simulink model "model_PD"  (R2016b)
settings: Solver=VariableStepAuto  StartTime=0.0  StopTime=30  FixedStep=Ts  RelTol=1e-3  EnableMultiTasking=on
values from neighbouring files (symbols this model uses):
  C = [eye(3),zeros(3,9);zeros(3,6),eye(3),zeros(3,3);zeros(3,9),eye(3)]    [model_script_Cascade.m]    (also in model_script_LQR_LQI.m; model_script_PD.m)
  D_height = .6117    (= 0.6117)    [model_script_Cascade.m]    (also in model_script_PD.m)
  D_pitch = .2256    (= 0.2256)    [model_script_Cascade.m]    (also in model_script_PD.m)
  D_roll = 0.1522    [model_script_Cascade.m]    (also in model_script_PD.m)
  D_yaw = .0367    (= 0.0367)    [model_script_Cascade.m]    (also in model_script_PD.m)
  g = 9.81    [model_script_Cascade.m]    (also in model_script_LQR_LQI.m; model_script_PD.m)
  I = diag([Ixx;Iyy;Izz])    [model_script_Cascade.m]    (also in model_script_LQR_LQI.m; model_script_PD.m)
  i0 = [tauphi;tautheta;taupsi;T]    [model_script_Cascade.m]    (also in model_script_LQR_LQI.m; model_script_PD.m)
  M = 0.487    [model_script_Cascade.m]    (also in model_script_LQR_LQI.m; model_script_PD.m)
  mean_att = zeros(3,1)    [model_script_Cascade.m]    (also in model_script_LQR_LQI.m; model_script_PD.m)
  mean_av = zeros(3,1)    [model_script_Cascade.m]    (also in model_script_LQR_LQI.m; model_script_PD.m)
  mean_pos = zeros(3,1)    [model_script_Cascade.m]    (also in model_script_LQR_LQI.m; model_script_PD.m)
  P_height = .3843    (= 0.3843)    [model_script_Cascade.m]    (also in model_script_PD.m)
  P_pitch = 1.9491    [model_script_Cascade.m]    (also in model_script_PD.m)
  P_roll = 1.5117    [model_script_Cascade.m]    (also in model_script_PD.m)
  P_yaw = .1152    (= 0.1152)    [model_script_Cascade.m]    (also in model_script_PD.m)
  propDistance = 0.125    [model_script_Cascade.m]    (also in model_script_LQR_LQI.m; model_script_PD.m)
  Q = diag([1e-5,1e-5,1e-5,1e-7,1e-7,1e-4,ones(1,2)*2e-7,6e-7,ones(1,3)*1e-7])    [model_script_Cascade.m]    (also in model_script_LQR_LQI.m; model_script_PD.m)
  R = diag(var)    [model_script_Cascade.m]    (also in model_script_LQR_LQI.m; model_script_PD.m)
  T_att = 1/200    (= 0.005)    [model_script_Cascade.m]    (also in model_script_LQR_LQI.m; model_script_PD.m)
  T_xy = 1/10    (= 0.1)    [model_script_Cascade.m]    (also in model_script_LQR_LQI.m; model_script_PD.m)
  T_yaw = 1/100    (= 0.01)    [model_script_Cascade.m]    (also in model_script_LQR_LQI.m; model_script_PD.m)
  T_z = 1/25    (= 0.04)    [model_script_Cascade.m]    (also in model_script_LQR_LQI.m; model_script_PD.m)
  var_att = [9.44454290406988e-06 1.41319492944844e-05 0.000590278082576831]'    [model_script_Cascade.m]    (also in model_script_LQR_LQI.m; model_script_PD.m)
  var_av = [8.38442613623844e-07 9.65548247114005e-07 1.06378940883219e-06]'    [model_script_Cascade.m]    (also in model_script_LQR_LQI.m; model_script_PD.m)
  var_pos = ones(3,1)*0.00219628793119666    [model_script_Cascade.m]    (also in model_script_LQR_LQI.m; model_script_PD.m)
  xi0 = [x;y;z;u;v;w;phi;theta;psi;p;q;r]    [model_script_Cascade.m]    (also in model_script_LQR_LQI.m; model_script_PD.m)
  yawTorqueC = 5    [model_script_Cascade.m]    (also in model_script_LQR_LQI.m; model_script_PD.m)
undefined symbols (not defined in the file or in its folder): den_phi_d, den_theta_d, den_z_d, num_phi_d, num_theta_d, num_z_d, sigbuilder_block, T_pos
undefined symbols (not defined in the file): dronePowerScaling
libraries: aerolibutil x2, simulink x2
(part 1 of 2)
settings Model: Creator=Patrick  LastModifiedBy=s122802
settings OptimizationCC: LifeSpan=inf
settings DebuggingCC: SFUnexpectedBacktrackingDiag=warning  SFNoUnconditionalDefaultTransitionDiag=warning  SFExecutionAtInitializationDiag=none
settings GRTTargetCC: TargetLangStandard=C89/C90 (ANSI)  GeneratePreprocessorConditionals=Disable all
settings ConfigComp: CovMetricSettings=dw  CovHtmlReporting=on  CovSaveCumulativeToWorkspaceVar=on  CovSaveSingleToWorkspaceVar=on  CovExternalEMLEnable=off

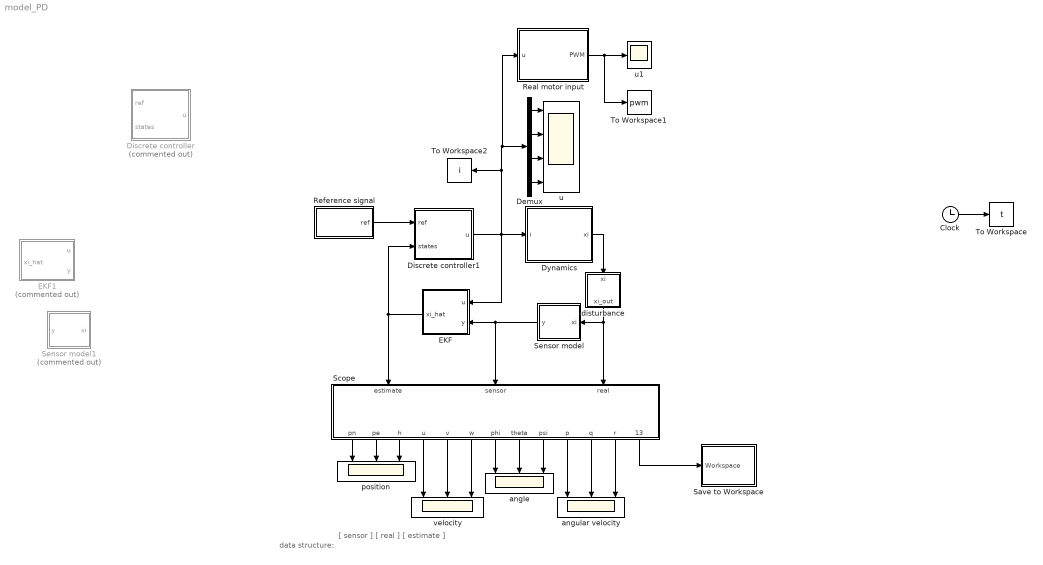
== system model_PD ==
  note: data structure:
  note: [ sensor   	]
      | [ real		]
      | [ estimate	]
  Clock : Clock
  Demux : Demux
  Discrete controller : Subsystem  Commented=on
  Discrete controller1 : Subsystem
  Dynamics : Subsystem
  EKF : Subsystem
  EKF1 : Subsystem  Commented=on
  Real motor input : Subsystem
  Reference signal : Subsystem
  Save to Workspace : Subsystem
  Scope : Subsystem
  Sensor model : Subsystem
  Sensor model1 : Subsystem  Commented=on
  To Workspace : ToWorkspace  VariableName=t  SampleTime=-1
      settings: Decimation=10
  To Workspace1 : ToWorkspace  VariableName=pwm  SampleTime=-1
      settings: Decimation=10
  To Workspace2 : ToWorkspace  VariableName=i  SampleTime=-1
      settings: Decimation=10
  angle : Scope  NumInputPorts=3
  angular velocity : Scope  NumInputPorts=3
  disturbance : Subsystem
  position : Scope  NumInputPorts=3
  u : Scope  NumInputPorts=4
  u1 : Scope
  velocity : Scope  NumInputPorts=3
  wires:
  Reference signal/1(ref) -> Discrete controller1/1(ref)
  Sensor model/1(y) -> EKF/2(y), Scope/2(sensor)
  Scope/2(pe) -> position/2
  Scope/10(p) -> angular velocity/1
  Scope/6(w) -> velocity/3
  Scope/5(v) -> velocity/2
  Scope/1(pn) -> position/1
  Scope/8(theta) -> angle/2
  Scope/9(psi) -> angle/3
  Scope/4(u) -> velocity/1
  Scope/11(q) -> angular velocity/2
  Scope/12(r) -> angular velocity/3
  Scope/3(h) -> position/3
  Dynamics/1(xi) -> disturbance/1(xi)
  EKF/1(xi_hat) -> Discrete controller1/2(states), Scope/1(estimate)
  Scope/13(Workspace) -> Save to Workspace/1(Workspace)
  Demux/1 -> u/1
  Demux/2 -> u/2
  Demux/3 -> u/3
  Demux/4 -> u/4
  Discrete controller1/1(u) -> EKF/1(u), To Workspace2/1, Real motor input/1(u), Demux/1, Dynamics/1(i)
  Scope/7(phi) -> angle/1
  disturbance/1(xi_out) -> Sensor model/1(xi), Scope/3(real)
  Real motor input/1(PWM) -> To Workspace1/1, u1/1
  Clock/1 -> To Workspace/1

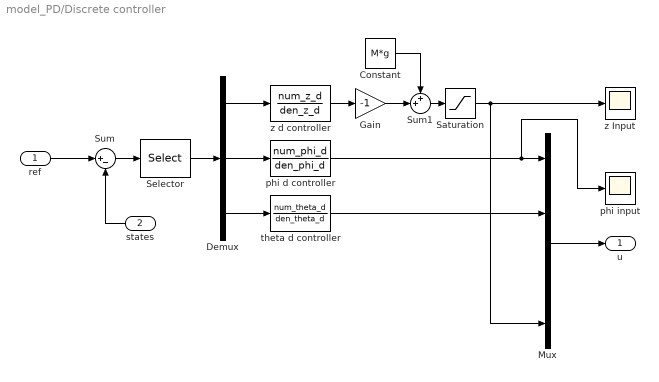
== system model_PD/Discrete controller ==
  ref : Inport
  states : Inport  Port=2
  Constant : Constant  Value=M*g
  Demux : Demux  Outputs=3
  Gain : Gain  Gain=-1
  Mux : Mux
  Saturation : Saturate  UpperLimit=10  LowerLimit=-10
  Selector : Selector  InputPortWidth=12  IndexOptions=Index vector (dialog)  Indices=[3 7 8]  OutputSizes=1
  Sum : Sum  Inputs=|+-
  Sum1 : Sum  Inputs=++|
  phi d controller : DiscreteTransferFcn  Numerator=num_phi_d  Denominator=den_phi_d
  phi input : Scope
  theta d controller : DiscreteTransferFcn  Numerator=num_theta_d  Denominator=den_theta_d
  z Input : Scope
  "z d controller " : DiscreteTransferFcn  Numerator=num_z_d  Denominator=den_z_d
  u : Outport
  wires:
  Demux/2 -> phi d controller/1
  Gain/1 -> Sum1/2
  Constant/1 -> Sum1/1
  Sum1/1 -> Saturation/1
  Selector/1 -> Demux/1
  Sum/1 -> Selector/1
  Demux/3 -> theta d controller/1
  Saturation/1 -> Mux/4, z Input/1
  "z d controller "/1 -> Gain/1
  theta d controller/1 -> Mux/2
  phi d controller/1 -> Mux/1, phi input/1
  states/1 -> Sum/2
  ref/1 -> Sum/1
  Demux/1 -> "z d controller "/1
  Mux/1 -> u/1

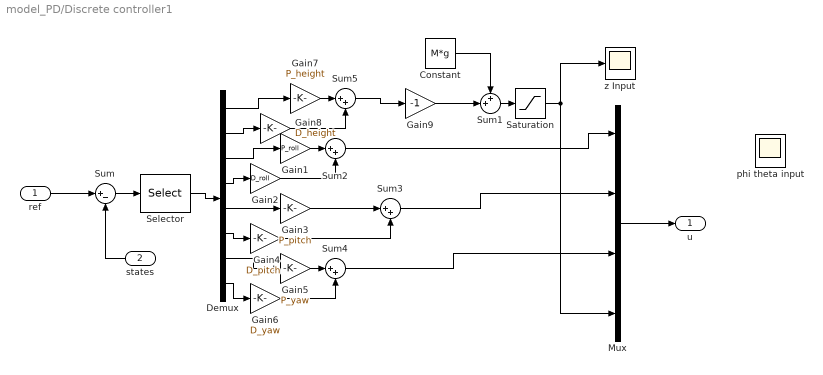
== system model_PD/Discrete controller1 ==
  ref : Inport
  states : Inport  Port=2
  Constant : Constant  Value=M*g
  Demux : Demux  Outputs=8
  Gain1 : Gain  Gain=P_roll
  Gain2 : Gain  Gain=D_roll
  Gain3 : Gain  Gain=P_pitch
  Gain4 : Gain  Gain=D_pitch
  Gain5 : Gain  Gain=P_yaw
  Gain6 : Gain  Gain=D_yaw
  Gain7 : Gain  Gain=P_height
  Gain8 : Gain  Gain=D_height
  Gain9 : Gain  Gain=-1
  Mux : Mux
  Saturation : Saturate  UpperLimit=10  LowerLimit=-10
  Selector : Selector  InputPortWidth=12  IndexOptions=Index vector (dialog)  Indices=[3 6 7 10 8 11 9 12]  OutputSizes=1
  Sum : Sum  Inputs=|+-
  Sum1 : Sum  Inputs=++|
  Sum{2..5} (4 alike) : Sum  Inputs=|++
  phi theta input : Scope  NumInputPorts=2
  z Input : Scope
  u : Outport
  wires:
  Mux/1 -> u/1
  ref/1 -> Sum/1
  states/1 -> Sum/2
  Sum3/1 -> Mux/2
  Saturation/1 -> Mux/4, z Input/1
  Sum/1 -> Selector/1
  Selector/1 -> Demux/1
  Sum1/1 -> Saturation/1
  Constant/1 -> Sum1/1
  Sum2/1 -> Mux/1
  Sum5/1 -> Gain9/1
  Gain5/1 -> Sum4/1
  Sum4/1 -> Mux/3
  Gain6/1 -> Sum4/2
  Gain2/1 -> Sum2/2
  Gain4/1 -> Sum3/2
  Gain1/1 -> Sum2/1
  Gain3/1 -> Sum3/1
  Demux/3 -> Gain1/1
  Demux/4 -> Gain2/1
  Demux/5 -> Gain3/1
  Demux/6 -> Gain4/1
  Demux/7 -> Gain5/1
  Demux/8 -> Gain6/1
  Gain8/1 -> Sum5/2
  Gain7/1 -> Sum5/1
  Demux/1 -> Gain7/1
  Demux/2 -> Gain8/1
  Gain9/1 -> Sum1/2

== system model_PD/Dynamics ==
  i : Inport
  Dynamics : Subsystem
  Mux : Mux
  xi : Outport
  wires:
  Mux/1 -> xi/1
  i/1 -> Dynamics/1(i)
  Dynamics/1(x y z) -> Mux/1
  Dynamics/2(u v w) -> Mux/2
  Dynamics/3(phi theta psi) -> Mux/3
  Dynamics/4(p q r) -> Mux/4

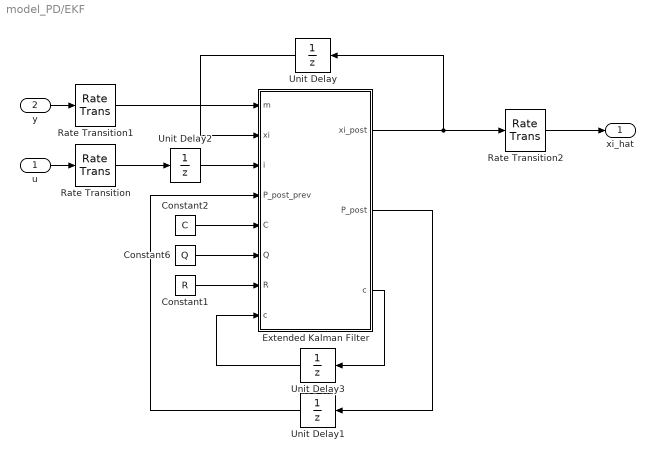
== system model_PD/EKF ==
  u : Inport
  y : Inport  Port=2
  Constant1 : Constant  Value=R
  Constant2 : Constant  Value=C
  Constant6 : Constant  Value=Q
  Extended Kalman Filter : MATLAB Function  TreatAsAtomicUnit=on
  Rate Transition : RateTransition  OutPortSampleTime=Ts
  Rate Transition1 : RateTransition  OutPortSampleTime=Ts
  Rate Transition2 : RateTransition  OutPortSampleTime=Ts
  Unit Delay : UnitDelay  InitialCondition=xi0  SampleTime=-1
  Unit Delay1 : UnitDelay  InitialCondition=zeros(12,12)  SampleTime=-1
  Unit Delay2 : UnitDelay  InitialCondition=i0  SampleTime=-1
  Unit Delay3 : UnitDelay  SampleTime=-1
  xi_hat : Outport
  wires:
  Extended Kalman Filter/3(c) -> Unit Delay3/1
  y/1 -> Rate Transition1/1
  Unit Delay3/1 -> Extended Kalman Filter/8("c ")
  Rate Transition2/1 -> xi_hat/1
  Rate Transition1/1 -> Extended Kalman Filter/1(m)
  Rate Transition/1 -> Unit Delay2/1
  u/1 -> Rate Transition/1
  Unit Delay2/1 -> Extended Kalman Filter/3(i)
  Unit Delay/1 -> Extended Kalman Filter/2(xi)
  Constant1/1 -> Extended Kalman Filter/7(R)
  Extended Kalman Filter/2(P_post) -> Unit Delay1/1
  Extended Kalman Filter/1(xi_post) -> Rate Transition2/1, Unit Delay/1
  Unit Delay1/1 -> Extended Kalman Filter/4(P_post_prev)
  Constant6/1 -> Extended Kalman Filter/6(Q)
  Constant2/1 -> Extended Kalman Filter/5(C)

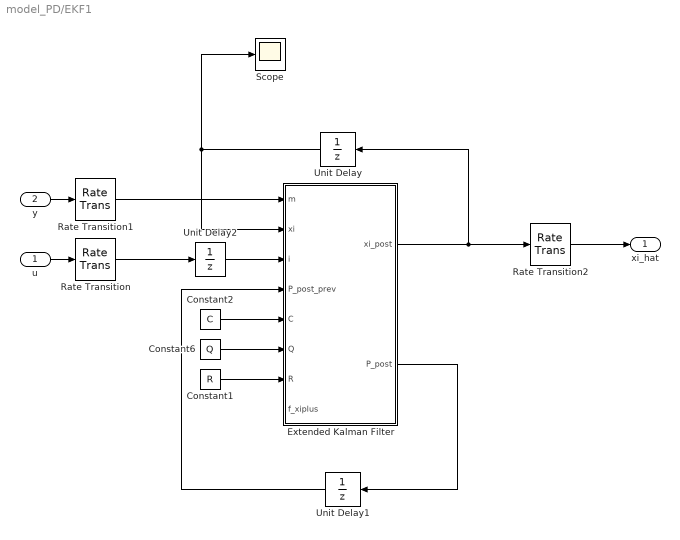
== system model_PD/EKF1 ==
  u : Inport
  y : Inport  Port=2
  Constant1 : Constant  Value=R
  Constant2 : Constant  Value=C
  Constant6 : Constant  Value=Q
  Extended Kalman Filter : MATLAB Function  TreatAsAtomicUnit=on
  Rate Transition : RateTransition  OutPortSampleTime=Ts
  Rate Transition1 : RateTransition  OutPortSampleTime=Ts
  Rate Transition2 : RateTransition  OutPortSampleTime=Ts
  Scope : Scope
  Unit Delay : UnitDelay  InitialCondition=xi0  SampleTime=-1
  Unit Delay1 : UnitDelay  InitialCondition=zeros(12,12)  SampleTime=-1
  Unit Delay2 : UnitDelay  InitialCondition=i0  SampleTime=-1
  xi_hat : Outport
  wires:
  Rate Transition2/1 -> xi_hat/1
  Rate Transition1/1 -> Extended Kalman Filter/1(m)
  Rate Transition/1 -> Unit Delay2/1
  y/1 -> Rate Transition1/1
  u/1 -> Rate Transition/1
  Unit Delay2/1 -> Extended Kalman Filter/3(i)
  Unit Delay/1 -> Extended Kalman Filter/2(xi), Scope/1
  Constant1/1 -> Extended Kalman Filter/7(R)
  Extended Kalman Filter/2(P_post) -> Unit Delay1/1
  Extended Kalman Filter/1(xi_post) -> Rate Transition2/1, Unit Delay/1
  Unit Delay1/1 -> Extended Kalman Filter/4(P_post_prev)
  Constant6/1 -> Extended Kalman Filter/6(Q)
  Constant2/1 -> Extended Kalman Filter/5(C)

== system model_PD/Real motor input ==
  u : Inport
  Constant : Constant  Value=100
  Demux : Demux
  Gain : Gain  Gain=0.25
  Motor input allocation Result is pure forces : Gain  Gain=[1 1/propDistance 1/propDistance -yawTorqueC; 1 -1/propDistance 1/propDistance yawTorqueC; 1 -1/propDistance -1/propDistance -yawTorqueC; 1 1/propDistance -1/propDistance yawTorqueC]  Multiplication=Matrix(K*u)  ParamDataTypeStr=int16
  Mux : Mux
  Newton To PWM : MATLAB Function  TreatAsAtomicUnit=on  mask{dronePowerScaling=dronePowerScaling}
      mask prompts: dronePowerScaling "Drone Power Factor"
  Saturation : Saturate  UpperLimit=100  LowerLimit=0.2
  Saturation Dynamic : simulink/Discontinuities/Saturation Dynamic  SCDEnableBlockLinearizationSpecification=on  OutMin=[]  OutMax=[]  OutDataTypeStr=Inherit: Same as second input  OutDataType=fixdt(1, 16)  OutScaling=2^-10  DoSatur=off
  throttleMinimum : Constant  Value=0
  PWM : Outport
  wires:
  throttleMinimum/1 -> Saturation Dynamic/3
  Constant/1 -> Saturation Dynamic/1
  Newton To PWM/1(PWM) -> Saturation Dynamic/2
  Motor input allocation Result is pure forces/1 -> Saturation/1
  Gain/1 -> Motor input allocation Result is pure forces/1
  Saturation/1 -> Newton To PWM/1(thrustIn)
  Saturation Dynamic/1 -> PWM/1
  u/1 -> Demux/1
  Demux/1 -> Mux/2
  Demux/2 -> Mux/3
  Demux/3 -> Mux/4
  Demux/4 -> Mux/1
  Mux/1 -> Gain/1

== system model_PD/Reference signal ==
  Mux : Mux  Inputs=12
  phi theta psi : Subsystem
  phi theta psi1 : Subsystem
  pn pe h : Subsystem
  u v w : Subsystem
  ref : Outport
  wires:
  pn pe h/1(pn) -> Mux/1
  pn pe h/2(pe) -> Mux/2
  pn pe h/3(h) -> Mux/3
  u v w/1(u) -> Mux/4
  u v w/2(v) -> Mux/5
  u v w/3(w) -> Mux/6
  phi theta psi/1(phi) -> Mux/7
  phi theta psi/2(theta) -> Mux/8
  phi theta psi/3(psi) -> Mux/9
  phi theta psi1/1(p) -> Mux/10
  phi theta psi1/2(q) -> Mux/11
  phi theta psi1/3(r) -> Mux/12
  Mux/1 -> ref/1

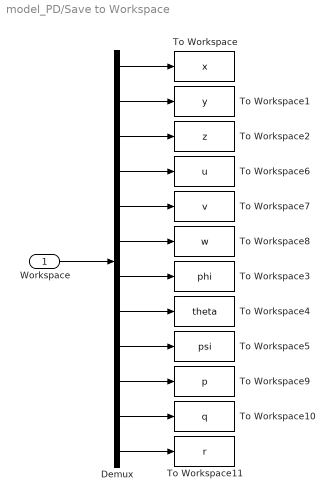
== system model_PD/Save to Workspace ==
  Workspace : Inport
  Demux : Demux  Outputs=12
  To Workspace : ToWorkspace  VariableName=x  SampleTime=-1
      settings: Decimation=10
  To Workspace1 : ToWorkspace  VariableName=y  SampleTime=-1
      settings: Decimation=10
  To Workspace10 : ToWorkspace  VariableName=q  SampleTime=-1
      settings: Decimation=10
  To Workspace11 : ToWorkspace  VariableName=r  SampleTime=-1
      settings: Decimation=10
  To Workspace2 : ToWorkspace  VariableName=z  SampleTime=-1
      settings: Decimation=10
  To Workspace3 : ToWorkspace  VariableName=phi  SampleTime=-1
      settings: Decimation=10
  To Workspace4 : ToWorkspace  VariableName=theta  SampleTime=-1
      settings: Decimation=10
  To Workspace5 : ToWorkspace  VariableName=psi  SampleTime=-1
      settings: Decimation=10
  To Workspace6 : ToWorkspace  VariableName=u  SampleTime=-1
      settings: Decimation=10
  To Workspace7 : ToWorkspace  VariableName=v  SampleTime=-1
      settings: Decimation=10
  To Workspace8 : ToWorkspace  VariableName=w  SampleTime=-1
      settings: Decimation=10
  To Workspace9 : ToWorkspace  VariableName=p  SampleTime=-1
      settings: Decimation=10
  wires:
  Workspace/1 -> Demux/1
  Demux/1 -> To Workspace/1
  Demux/2 -> To Workspace1/1
  Demux/3 -> To Workspace2/1
  Demux/4 -> To Workspace6/1
  Demux/5 -> To Workspace7/1
  Demux/6 -> To Workspace8/1
  Demux/7 -> To Workspace3/1
  Demux/8 -> To Workspace4/1
  Demux/10 -> To Workspace9/1
  Demux/9 -> To Workspace5/1
  Demux/11 -> To Workspace10/1
  Demux/12 -> To Workspace11/1

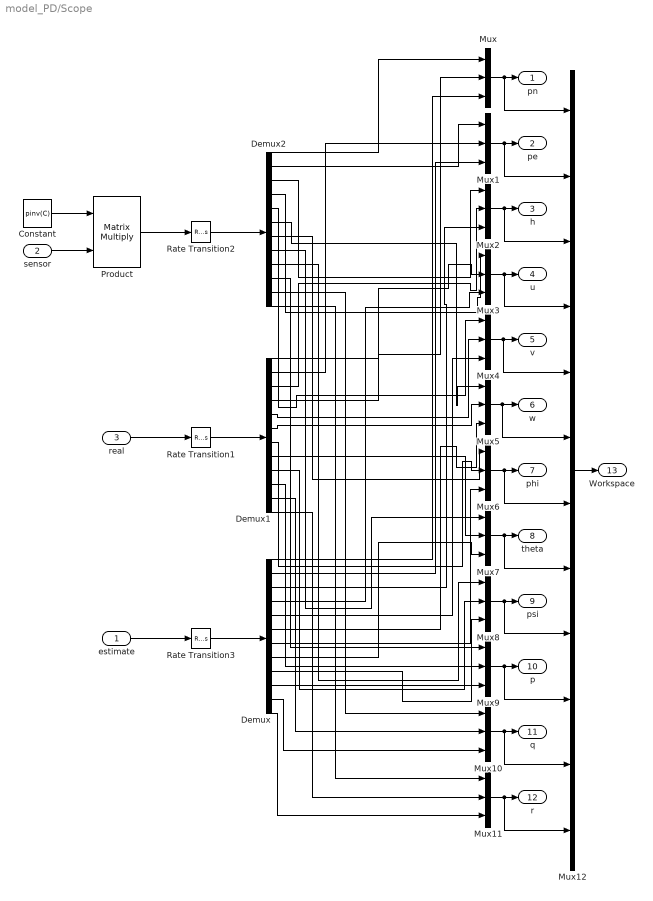
== system model_PD/Scope ==
  estimate : Inport
  sensor : Inport  Port=2
  real : Inport  Port=3
  Constant : Constant  Value=pinv(C)
  Demux : Demux  Outputs=12
  Demux1 : Demux  Outputs=12
  Demux2 : Demux  Outputs=12
  Mux{,1..11} (12 alike) : Mux  Inputs=3
  Mux12 : Mux  Inputs=12
  Product : Product  Multiplication=Matrix(*)
  Rate Transition1 : RateTransition  OutPortSampleTime=Ts
  Rate Transition2 : RateTransition  OutPortSampleTime=Ts
  Rate Transition3 : RateTransition  OutPortSampleTime=Ts
  pn : Outport
  pe : Outport  Port=2
  h : Outport  Port=3
  u : Outport  Port=4
  v : Outport  Port=5
  w : Outport  Port=6
  phi : Outport  Port=7
  theta : Outport  Port=8
  psi : Outport  Port=9
  p : Outport  Port=10
  q : Outport  Port=11
  r : Outport  Port=12
  Workspace : Outport  Port=13
  wires:
  Demux2/1 -> Mux/1
  Demux1/1 -> Mux/2
  Demux/1 -> Mux/3
  Demux2/2 -> Mux1/1
  Demux1/2 -> Mux1/2
  Demux/2 -> Mux1/3
  Demux2/3 -> Mux2/1
  Demux1/3 -> Mux2/2
  Demux/3 -> Mux2/3
  Mux/1 -> Mux12/1, pn/1
  Mux1/1 -> Mux12/2, pe/1
  Demux2/4 -> Mux3/1
  Demux1/4 -> Mux3/2
  Demux/4 -> Mux3/3
  Mux3/1 -> Mux12/4, u/1
  Demux2/5 -> Mux4/1
  Demux1/5 -> Mux4/2
  Demux/5 -> Mux4/3
  Mux4/1 -> Mux12/5, v/1
  Demux2/6 -> Mux5/1
  Demux1/6 -> Mux5/2
  Demux/6 -> Mux5/3
  Mux5/1 -> Mux12/6, w/1
  Mux6/1 -> Mux12/7, phi/1
  Demux2/7 -> Mux6/1
  Demux1/7 -> Mux6/2
  Demux/7 -> Mux6/3
  Mux7/1 -> Mux12/8, theta/1
  Demux2/8 -> Mux7/1
  Demux1/8 -> Mux7/2
  Demux/8 -> Mux7/3
  Mux8/1 -> Mux12/9, psi/1
  Demux2/9 -> Mux8/1
  Demux1/9 -> Mux8/2
  Demux/9 -> Mux8/3
  Mux9/1 -> Mux12/10, p/1
  Mux10/1 -> Mux12/11, q/1
  Mux11/1 -> Mux12/12, r/1
  Demux2/10 -> Mux9/1
  Demux1/10 -> Mux9/2
  Demux/10 -> Mux9/3
  Demux2/11 -> Mux10/1
  Demux1/11 -> Mux10/2
  Demux/11 -> Mux10/3
  Demux2/12 -> Mux11/1
  Demux1/12 -> Mux11/2
  Demux/12 -> Mux11/3
  estimate/1 -> Rate Transition3/1
  Mux2/1 -> Mux12/3, h/1
  Mux12/1 -> Workspace/1
  sensor/1 -> Product/2
  Product/1 -> Rate Transition2/1
  Constant/1 -> Product/1
  Rate Transition2/1 -> Demux2/1
  Rate Transition1/1 -> Demux1/1
  Rate Transition3/1 -> Demux/1
  real/1 -> Rate Transition1/1

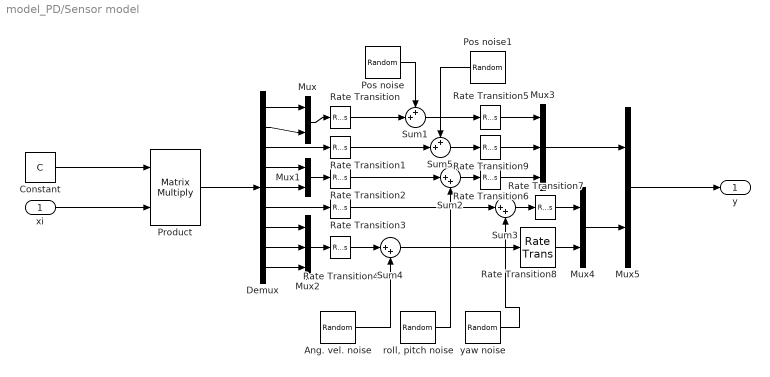
== system model_PD/Sensor model ==
  xi : Inport
  Ang. vel. noise : RandomNumber  Mean=mean_av  Variance=var_av  Seed=[7;8;9]  SampleTime=T_yaw  VectorParams1D=off
  Constant : Constant  Value=C
  Demux : Demux  Outputs=9
  Mux{,1,4..5} (4 alike) : Mux  Inputs=2
  Mux2 : Mux  Inputs=3
  Mux3 : Mux  Inputs=3
  Pos noise : RandomNumber  Mean=mean_pos(1:2)  Variance=var_pos(1:2)  Seed=[1;2]  SampleTime=T_xy  VectorParams1D=off
  Pos noise1 : RandomNumber  Mean=mean_pos(3)  Variance=var_pos(3)  Seed=3  SampleTime=T_z  VectorParams1D=off
  Product : Product  Multiplication=Matrix(*)
  Rate Transition : RateTransition  OutPortSampleTime=T_xy
  Rate Transition1 : RateTransition  OutPortSampleTime=T_z
  Rate Transition2 : RateTransition  OutPortSampleTime=T_att
  Rate Transition3 : RateTransition  OutPortSampleTime=T_yaw
  Rate Transition4 : RateTransition  OutPortSampleTime=T_yaw
  Rate Transition{5..9} (5 alike) : RateTransition  OutPortSampleTime=Ts
  Sum1 : Sum  Inputs=++|
  Sum2 : Sum  Inputs=|++
  Sum3 : Sum  Inputs=|++
  Sum4 : Sum  Inputs=|++
  Sum5 : Sum  Inputs=++|
  "roll, pitch noise" : RandomNumber  Mean=mean_att(1:2)  Variance=var_att(1:2)  Seed=[4;5]  SampleTime=T_att  VectorParams1D=off
  yaw noise : RandomNumber  Mean=mean_att(3,1)  Variance=var_att(3,1)  Seed=6  SampleTime=T_yaw  VectorParams1D=off
  y : Outport
  wires:
  Rate Transition9/1 -> Mux3/2
  Rate Transition1/1 -> Sum5/2
  Sum5/1 -> Rate Transition9/1
  Pos noise1/1 -> Sum5/1
  Rate Transition6/1 -> Mux3/3
  Rate Transition8/1 -> Mux4/2
  Rate Transition7/1 -> Mux4/1
  Rate Transition5/1 -> Mux3/1
  Mux5/1 -> y/1
  Rate Transition4/1 -> Sum4/1
  Rate Transition3/1 -> Sum3/1
  Rate Transition2/1 -> Sum2/1
  Rate Transition/1 -> Sum1/2
  Mux4/1 -> Mux5/2
  Mux3/1 -> Mux5/1
  Sum4/1 -> Rate Transition8/1
  Sum3/1 -> Rate Transition7/1
  Sum2/1 -> Rate Transition6/1
  Sum1/1 -> Rate Transition5/1
  Mux2/1 -> Rate Transition4/1
  Demux/9 -> Mux2/3
  Demux/8 -> Mux2/2
  Demux/7 -> Mux2/1
  Demux/6 -> Rate Transition3/1
  Mux1/1 -> Rate Transition2/1
  Mux/1 -> Rate Transition/1
  Pos noise/1 -> Sum1/1
  Demux/5 -> Mux1/2
  Demux/4 -> Mux1/1
  Demux/1 -> Mux/1
  Demux/2 -> Mux/2
  Demux/3 -> Rate Transition1/1
  Product/1 -> Demux/1
  Ang. vel. noise/1 -> Sum4/2
  yaw noise/1 -> Sum3/2
  "roll, pitch noise"/1 -> Sum2/2
  Constant/1 -> Product/1
  xi/1 -> Product/2

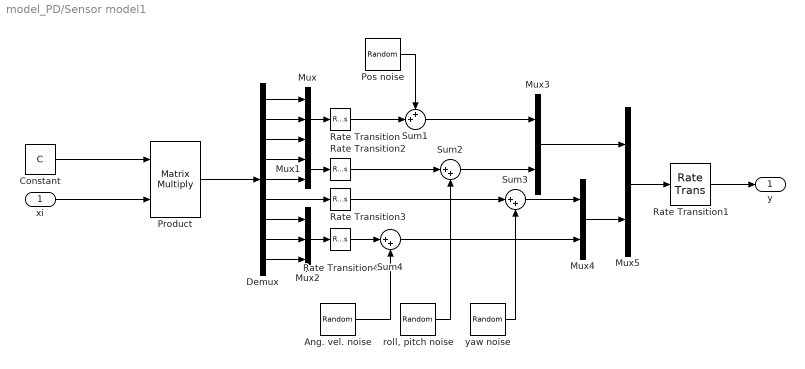
== system model_PD/Sensor model1 ==
  xi : Inport
  Ang. vel. noise : RandomNumber  Mean=mean_av  Variance=var_av  Seed=[7;8;9]  SampleTime=T_yaw  VectorParams1D=off
  Constant : Constant  Value=C
  Demux : Demux  Outputs=9
  Mux : Mux  Inputs=3
  Mux{1,3..5} (4 alike) : Mux  Inputs=2
  Mux2 : Mux  Inputs=3
  Pos noise : RandomNumber  Mean=mean_pos  Variance=var_pos  Seed=[1;2;3]  SampleTime=T_pos  VectorParams1D=off
  Product : Product  Multiplication=Matrix(*)
  Rate Transition : RateTransition  OutPortSampleTime=T_pos
  Rate Transition1 : RateTransition  OutPortSampleTime=Ts
  Rate Transition2 : RateTransition  OutPortSampleTime=T_att
  Rate Transition3 : RateTransition  OutPortSampleTime=T_yaw
  Rate Transition4 : RateTransition  OutPortSampleTime=T_yaw
  Sum1 : Sum  Inputs=++|
  Sum2 : Sum  Inputs=|++
  Sum3 : Sum  Inputs=|++
  Sum4 : Sum  Inputs=|++
  "roll, pitch noise" : RandomNumber  Mean=mean_att(1:2)  Variance=var_att(1:2)  Seed=[4;5]  SampleTime=T_att  VectorParams1D=off
  yaw noise : RandomNumber  Mean=mean_att(3,1)  Variance=var_att(3,1)  Seed=6  SampleTime=T_yaw  VectorParams1D=off
  y : Outport
  wires:
  Rate Transition1/1 -> y/1
  Rate Transition4/1 -> Sum4/1
  Rate Transition3/1 -> Sum3/1
  Rate Transition2/1 -> Sum2/1
  Rate Transition/1 -> Sum1/2
  Mux5/1 -> Rate Transition1/1
  Mux4/1 -> Mux5/2
  Mux3/1 -> Mux5/1
  Sum4/1 -> Mux4/2
  Sum3/1 -> Mux4/1
  Sum2/1 -> Mux3/2
  Sum1/1 -> Mux3/1
  Mux2/1 -> Rate Transition4/1
  Demux/9 -> Mux2/3
  Demux/8 -> Mux2/2
  Demux/7 -> Mux2/1
  Demux/6 -> Rate Transition3/1
  Mux1/1 -> Rate Transition2/1
  Mux/1 -> Rate Transition/1
  Pos noise/1 -> Sum1/1
  Demux/5 -> Mux1/2
  Demux/4 -> Mux1/1
  Demux/1 -> Mux/1
  Demux/2 -> Mux/2
  Demux/3 -> Mux/3
  Product/1 -> Demux/1
  Ang. vel. noise/1 -> Sum4/2
  yaw noise/1 -> Sum3/2
  "roll, pitch noise"/1 -> Sum2/2
  Constant/1 -> Product/1
  xi/1 -> Product/2

== system model_PD/disturbance ==
  note: x
  note: y
  note: z
  note: u
  note: v
  note: w
  note: phi
  note: theta
  note: psi
  note: p
  note: q
  note: r
  xi : Inport
  Demux : Demux  Outputs=12
  Mux : Mux  Inputs=12
  Signal Builder : Subsystem  Tag=STV Subsys  LoadFcn=sigbuilder_block('load');  StartFcn=sigbuilder_block('start');  StopFcn=sigbuilder_block('stop');  ClipboardFcn=sigbuilder_block('clipboard');  mask(Sigbuilder block){tuvar=[0:10]}
      mask help: Simulink:masks:SigbuilderBlock_MD
      mask init:
      | if ~strcmp(get_param(bdroot(gcbh),'SimulationStatus'),'stopped') tuvar = sigbuilder_block('maskInit'); end
      settings: CopyFcn=sigbuilder_block('copy');  DeleteFcn=sigbuilder_block('delete');  ModelCloseFcn=sigbuilder_block('modelClose');  PreSaveFcn=sigbuilder_block('preSave');  PauseFcn=sigbuilder_block('pause');  ContinueFcn=sigbuilder_block('continue');  NameChangeFcn=sigbuilder_block('namechange');  OpenFcn=sigbuilder_block('open',[437.6 199.2 550.4 400 ]);  CloseFcn=sigbuilder_block('close');
      mask Display: plot(0, 0, 100, 100,[2, 2, 32, 32, 2], [68, 8, 8, 68, 68],[32, 2], [38, 38], [32, 19, 2],[53, 60, 44], [32, 17, 17, 2],[16, 16, 31, 31]);txt = getActiveGroup(gcbh);text(2, 100, txt,'verticalAlignment', 'top');
  Sum : Sum  Inputs=|++
  xi_out : Outport
  wires:
  Signal Builder/1(Signal 1) -> Sum/2
  Sum/1 -> Mux/7
  Demux/7 -> Sum/1
  Mux/1 -> xi_out/1
  Demux/10 -> Mux/10
  Demux/9 -> Mux/9
  Demux/8 -> Mux/8
  Demux/6 -> Mux/6
  Demux/5 -> Mux/5
  Demux/4 -> Mux/4
  Demux/3 -> Mux/3
  Demux/2 -> Mux/2
  Demux/1 -> Mux/1
  Demux/11 -> Mux/11
  Demux/12 -> Mux/12
  xi/1 -> Demux/1

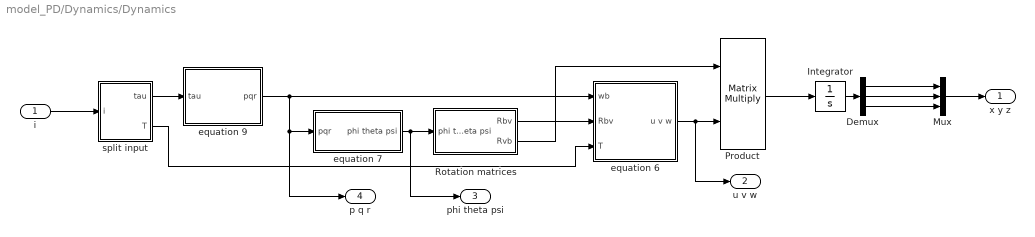
== system model_PD/Dynamics/Dynamics ==
  i : Inport
  Demux : Demux  Outputs=3
  Integrator : Integrator  InitialCondition=[0;0;0]
  Mux : Mux  Inputs=3
  Product : Product  Multiplication=Matrix(*)
  Rotation matrices : Subsystem
  equation 6 : Subsystem
  equation 7 : Subsystem
  equation 9 : Subsystem
  split input : Subsystem
  x y z : Outport
  u v w : Outport  Port=2
  phi theta psi : Outport  Port=3
  p q r : Outport  Port=4
  wires:
  Product/1 -> Integrator/1
  Rotation matrices/2(Rvb) -> Product/1
  equation 9/1(pqr) -> equation 7/1(pqr), p q r/1, equation 6/1(wb)
  equation 7/1(phi theta psi) -> Rotation matrices/1(phi theta psi), phi theta psi/1
  equation 6/1(u v w) -> u v w/1, Product/2
  Rotation matrices/1(Rbv) -> equation 6/2(Rbv)
  i/1 -> split input/1(i)
  split input/1(tau) -> equation 9/1(tau)
  split input/2(T) -> equation 6/3(T)
  Integrator/1 -> Demux/1
  Demux/2 -> Mux/2
  Demux/1 -> Mux/1
  Mux/1 -> x y z/1
  Demux/3 -> Mux/3

== system model_PD/Reference signal/phi theta psi ==
  Constant1 : Constant  Value=0
  Constant2 : Constant  Value=0
  Constant3 : Constant  Value=0
  phi : Outport
  theta : Outport  Port=2
  psi : Outport  Port=3
  wires:
  Constant3/1 -> psi/1
  Constant1/1 -> phi/1
  Constant2/1 -> theta/1

== system model_PD/Reference signal/phi theta psi1 ==
  Constant1 : Constant  Value=0
  Constant2 : Constant  Value=0
  Constant3 : Constant  Value=0
  p : Outport
  q : Outport  Port=2
  r : Outport  Port=3
  wires:
  Constant1/1 -> p/1
  Constant2/1 -> q/1
  Constant3/1 -> r/1

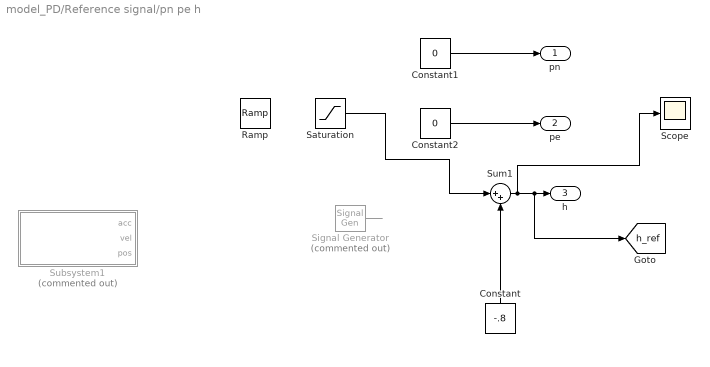
== system model_PD/Reference signal/pn pe h ==
  Constant : Constant  Value=-.8
  Constant1 : Constant  Value=0
  Constant2 : Constant  Value=0
  Ramp : simulink/Sources/Ramp  slope=-0.1  start=0  X0=0
  Saturation : Saturate  UpperLimit=0  LowerLimit=-1
  Scope : Scope
  Signal Generator : SignalGenerator  Commented=on  WaveForm=square  Amplitude=.2  Frequency=.2  Units=rad/sec
  Subsystem1 : Subsystem  Commented=on  mask(Ref3){}
      settings: OpenFcn=r3g_main
      mask Display: disp('Ref3');
  Sum1 : Sum  Inputs=|++
  pn : Outport
  pe : Outport  Port=2
  h : Outport  Port=3
  tag scope: h_ref=global
  wires:
  Signal Generator/1 -> ?
  Sum1/1 -> Scope/1, [h_ref], h/1
  Constant/1 -> Sum1/2
  Constant2/1 -> pe/1
  Constant1/1 -> pn/1
  Saturation/1 -> Sum1/1

== system model_PD/Reference signal/u v w ==
  Constant1 : Constant  Value=0
  Constant2 : Constant  Value=0
  Constant3 : Constant  Value=0
  u : Outport
  v : Outport  Port=2
  w : Outport  Port=3
  wires:
  Constant3/1 -> w/1
  Constant1/1 -> u/1
  Constant2/1 -> v/1

== system model_PD/disturbance/Signal Builder ==
  Demux : Demux  Tag=STV Demux  Outputs=1
  FromWs : FromWorkspace  Tag=STV FromWs  VariableName=tuvar  SampleTime=0
      SigBuilderData=|
      | common.afterFinalStr = 'Extrapolate'
      | common.sampleTime = 0
      | dataSet.timeRange = [0 30]
      | dataSet.name = 'Group 1'
      | sbobj.Groups.Name = 'Group 1'
      | sbobj.Groups.Signals.Name = 'Signal 1'
      | sbobj.Groups.Signals.XData = [0 11.1 11.1 12.35 12.35 30]
      | sbobj.Groups.Signals.YData = [0 0 0.02 0.02 0 0]
      | sbobj.Groups.TimeRange = [0 30]
  Signal 1 : Outport  Tag=STV Outport
  wires:
  FromWs/1 -> Demux/1
  Demux/1 -> Signal 1/1

== system model_PD/Dynamics/Dynamics/Rotation matrices ==
  phi theta psi : Inport
  Rotm in euler : MATLAB Function  TreatAsAtomicUnit=on
  Transpose : Math  Operator=transpose  SaturateOnIntegerOverflow=on
  Rbv : Outport
  Rvb : Outport  Port=2
  wires:
  phi theta psi/1 -> Rotm in euler/1(alpha)
  Rotm in euler/1(Rbv) -> Rbv/1, Transpose/1
  Transpose/1 -> Rvb/1

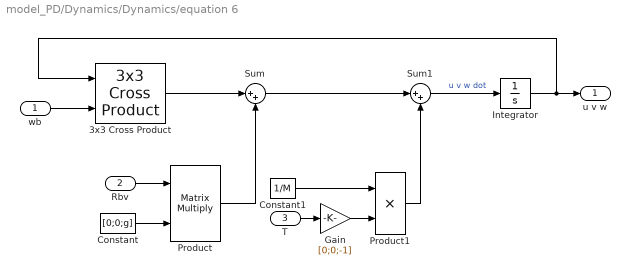
== system model_PD/Dynamics/Dynamics/equation 6 ==
  wb : Inport
  Rbv : Inport  Port=2
  T : Inport  Port=3
  3x3 Cross Product : aerolibutil/3x3 Cross Product
  Constant : Constant  Value=[0;0;g]
  Constant1 : Constant  Value=1/M
  Gain : Gain  Gain=[0;0;-1]
  Integrator : Integrator
  Product : Product  Multiplication=Matrix(*)
  Product1 : Product
  Sum : Sum  Inputs=|++
  Sum1 : Sum  Inputs=|++
  u v w : Outport
  wires:
  3x3 Cross Product/1 -> Sum/1
  wb/1 -> 3x3 Cross Product/2
  Product/1 -> Sum/2
  Rbv/1 -> Product/1
  Constant/1 -> Product/2
  Sum/1 -> Sum1/1
  Product1/1 -> Sum1/2
  Constant1/1 -> Product1/1
  T/1 -> Gain/1
  Sum1/1 -> Integrator/1  "u v w dot"
  Integrator/1 -> 3x3 Cross Product/1, u v w/1
  Gain/1 -> Product1/2

== system model_PD/Dynamics/Dynamics/equation 7 ==
  pqr : Inport
  Integrator : Integrator  InitialCondition=[0;0;0]
  MATLAB Function : MATLAB Function  TreatAsAtomicUnit=on
  Product : Product  Multiplication=Matrix(*)
  phi theta psi : Outport
  wires:
  MATLAB Function/1(E) -> Product/1
  pqr/1 -> Product/2
  Product/1 -> Integrator/1  "phi theta psi dot"
  Integrator/1 -> phi theta psi/1, MATLAB Function/1(alpha)

== system model_PD/Dynamics/Dynamics/equation 9 ==
  tau : Inport
  3x3 Cross Product : aerolibutil/3x3 Cross Product
  Constant : Constant  Value=I
  Divide : Product  Inputs=/  Multiplication=Matrix(*)
  Integrator : Integrator
  Product : Product  Multiplication=Matrix(*)
  Product1 : Product  Multiplication=Matrix(*)
  Sum : Sum  Inputs=|++
  pqr : Outport
  wires:
  Constant/1 -> Product1/1, Divide/1
  Sum/1 -> Product/2
  tau/1 -> Sum/2
  3x3 Cross Product/1 -> Sum/1
  Product1/1 -> 3x3 Cross Product/1
  Divide/1 -> Product/1
  Integrator/1 -> pqr/1, 3x3 Cross Product/2, Product1/2
  Product/1 -> Integrator/1  "pqr dot"

== system model_PD/Dynamics/Dynamics/split input ==
  i : Inport
  Demux : Demux
  Mux : Mux  Inputs=3
  tau : Outport
  T : Outport  Port=2
  wires:
  Demux/2 -> Mux/2
  Demux/3 -> Mux/3
  i/1 -> Demux/1
  Mux/1 -> tau/1
  Demux/4 -> T/1
  Demux/1 -> Mux/1

== system model_PD/Reference signal/pn pe h/Subsystem1 ==
  Constant : Constant
  Demux : Demux  Outputs=3
  S-Function : S-Function  FunctionName=ref3  Parameters=ref_part  SFunctionDeploymentMode=off  EnableBusSupport=off
      settings: OpenFcn=global ref_part; r3g_main
  acc : Outport
  vel : Outport  Port=2
  pos : Outport  Port=3
  wires:
  Constant/1 -> S-Function/1
  S-Function/1 -> Demux/1
  Demux/1 -> acc/1
  Demux/2 -> vel/1
  Demux/3 -> pos/1

== matlab function model_PD/EKF1/Extended Kalman Filter ==
  data: m input; xi input; i input; P_post_prev input; xi_post output; C input; Q input; R input; P_post output; f_xiplus input
function [xi_post,P_post] = fcn(m,xi,i,P_post_prev,C,Q,R,f_xiplus)
%% Prediction
x = xi(1);      y     = xi(2);      z   = xi(3);
u = xi(4);      v     = xi(5);      w   = xi(6);
phi = xi(7);    theta = xi(8);      psi = xi(9);
p   = xi(10);   q     = xi(11);     r   = xi(12);

tauphi = i(1);  tautheta = i(2);
taupsi = i(3);  T = i(4);

xi_prio = ...
[x - (v*(cos(conj(phi))*sin(conj(psi)) - cos(conj(psi))*sin(conj(phi))*sin(conj(theta))))/400 + (w*(sin(conj(phi))*sin(conj(psi)) + cos(conj(phi))*cos(conj(psi))*sin(conj(theta))))/400 + (u*cos(conj(psi))*cos(conj(theta)))/400;
 y + (v*(cos(conj(phi))*cos(conj(psi)) + sin(conj(phi))*sin(conj(psi))*sin(conj(theta))))/400 - (w*(cos(conj(psi))*sin(conj(phi)) - cos(conj(phi))*sin(conj(psi))*sin(conj(theta))))/400 + (u*cos(conj(theta))*sin(conj(psi)))/400;
                                                                                                                  z - (u*sin(conj(theta)))/400 + (w*cos(conj(phi))*cos(conj(theta)))/400 + (v*cos(conj(theta))*sin(conj(phi)))/400;
                                                                                                                                                                                u - (981*sin(theta))/40000 - (q*w)/400 + (r*v)/400;
                                                                                                                                                                       v + (981*cos(theta)*sin(phi))/40000 + (p*w)/400 - (r*u)/400;
                                                                                                                                                           w - (5*T)/974 + (981*cos(phi)*cos(theta))/40000 - (p*v)/400 + (q*u)/400;
                                                                                                                                                           p/400 + phi + (r*cos(phi)*tan(theta))/400 + (q*sin(phi)*tan(theta))/400;
                                                                                                                                                                                       theta + (q*cos(phi))/400 - (r*sin(phi))/400;
                                                                                                                                                               psi + (r*cos(phi))/(400*cos(theta)) + (q*sin(phi))/(400*cos(theta));
                                                                                                                                                                                                  p + (5*tauphi)/4 - (43*q*r)/8000;
                                                                                                                                                                                              q + (25*tautheta)/16 + (39*p*r)/6400;
                                                                                                                                                                                                   r + (25*taupsi)/59 + (p*q)/5900];

A = ...
[1, 0, 0, (cos(conj(psi))*cos(conj(theta)))/400, (cos(conj(psi))*sin(conj(phi))*sin(conj(theta)))/400 - (cos(conj(phi))*sin(conj(psi)))/400, (sin(conj(phi))*sin(conj(psi)))/400 + (cos(conj(phi))*cos(conj(psi))*sin(conj(theta)))/400,   (v*(sin(conj(phi))*sin(conj(psi)) + cos(conj(phi))*cos(conj(psi))*sin(conj(theta))))/400 + (w*(cos(conj(phi))*sin(conj(psi)) - cos(conj(psi))*sin(conj(phi))*sin(conj(theta))))/400, (w*cos(conj(phi))*cos(conj(psi))*cos(conj(theta)))/400 - (u*cos(conj(psi))*sin(conj(theta)))/400 + (v*cos(conj(psi))*cos(conj(theta))*sin(conj(phi)))/400, (w*(cos(conj(psi))*sin(conj(phi)) - cos(conj(phi))*sin(conj(psi))*sin(conj(theta))))/400 - (v*(cos(conj(phi))*cos(conj(psi)) + sin(conj(phi))*sin(conj(psi))*sin(conj(theta))))/400 - (u*cos(conj(theta))*sin(conj(psi)))/400,           0,                         0,                         0;
 0, 1, 0, (cos(conj(theta))*sin(conj(psi)))/400, (cos(conj(phi))*cos(conj(psi)))/400 + (sin(conj(phi))*sin(conj(psi))*sin(conj(theta)))/400, (cos(conj(phi))*sin(conj(psi))*sin(conj(theta)))/400 - (cos(conj(psi))*sin(conj(phi)))/400, - (v*(cos(conj(psi))*sin(conj(phi)) - cos(conj(phi))*sin(conj(psi))*sin(conj(theta))))/400 - (w*(cos(conj(phi))*cos(conj(psi)) + sin(conj(phi))*sin(conj(psi))*sin(conj(theta))))/400, (w*cos(conj(phi))*cos(conj(theta))*sin(conj(psi)))/400 - (u*sin(conj(psi))*sin(conj(theta)))/400 + (v*cos(conj(theta))*sin(conj(phi))*sin(conj(psi)))/400, (w*(sin(conj(phi))*sin(conj(psi)) + cos(conj(phi))*cos(conj(psi))*sin(conj(theta))))/400 - (v*(cos(conj(phi))*sin(conj(psi)) - cos(conj(psi))*sin(conj(phi))*sin(conj(theta))))/400 + (u*cos(conj(psi))*cos(conj(theta)))/400,           0,                         0,                         0;
 0, 0, 1,                 -sin(conj(theta))/400,                                                      (cos(conj(theta))*sin(conj(phi)))/400,                                                      (cos(conj(phi))*cos(conj(theta)))/400,                                                                                                     (v*cos(conj(phi))*cos(conj(theta)))/400 - (w*cos(conj(theta))*sin(conj(phi)))/400,                                            - (u*cos(conj(theta)))/400 - (w*cos(conj(phi))*sin(conj(theta)))/400 - (v*sin(conj(phi))*sin(conj(theta)))/400,                                                                                                                                                                                                                             0,           0,                         0,                         0;
 0, 0, 0,                                     1,                                                                                      r/400,                                                                                     -q/400,                                                                                                                                                                                     0,                                                                                                                                   -(981*cos(theta))/40000,                                                                                                                                                                                                                             0,           0,                    -w/400,                     v/400;
 0, 0, 0,                                -r/400,                                                                                          1,                                                                                      p/400,                                                                                                                                                       (981*cos(phi)*cos(theta))/40000,                                                                                                                          -(981*sin(phi)*sin(theta))/40000,                                                                                                                                                                                                                             0,       w/400,                         0,                    -u/400;
 0, 0, 0,                                 q/400,                                                                                     -p/400,                                                                                          1,                                                                                                                                                      -(981*cos(theta)*sin(phi))/40000,                                                                                                                          -(981*cos(phi)*sin(theta))/40000,                                                                                                                                                                                                                             0,      -v/400,                     u/400,                         0;
 0, 0, 0,                                     0,                                                                                          0,                                                                                          0,                                                                                                                         (q*cos(phi)*tan(theta))/400 - (r*sin(phi)*tan(theta))/400 + 1,                                                                                 (r*cos(phi)*(tan(theta)^2 + 1))/400 + (q*sin(phi)*(tan(theta)^2 + 1))/400,                                                                                                                                                                                                                             0,       1/400, (sin(phi)*tan(theta))/400, (cos(phi)*tan(theta))/400;
 0, 0, 0,                                     0,                                                                                          0,                                                                                          0,                                                                                                                                                 - (r*cos(phi))/400 - (q*sin(phi))/400,                                                                                                                                                         1,                                                                                                                                                                                                                             0,           0,              cos(phi)/400,             -sin(phi)/400;
 0, 0, 0,                                     0,                                                                                          0,                                                                                          0,                                                                                                                         (q*cos(phi))/(400*cos(theta)) - (r*sin(phi))/(400*cos(theta)),                                                                   (r*cos(phi)*sin(theta))/(400*cos(theta)^2) + (q*sin(phi)*sin(theta))/(400*cos(theta)^2),                                                                                                                                                                                                                             1,           0, sin(phi)/(400*cos(theta)), cos(phi)/(400*cos(theta));
 0, 0, 0,                                     0,                                                                                          0,                                                                                          0,                                                                                                                                                                                     0,                                                                                                                                                         0,                                                                                                                                                                                                                             0,           1,              -(43*r)/8000,              -(43*q)/8000;
 0, 0, 0,                                     0,                                                                                          0,                                                                                          0,                                                                                                                                                                                     0,                                                                                                                                                         0,                                                                                                                                                                                                                             0, (39*r)/6400,                         1,               (39*p)/6400;
 0, 0, 0,                                     0,                                                                                          0,                                                                                          0,                                                                                                                                                                                     0,                                                                                                                                                         0,                                                                                                                                                                                                                             0,      q/5900,                    p/5900,                         1];

P_prio = A*P_post_prev*A'+Q;

%% Update
K = P_prio*C'/(C*P_prio*C'+R);
xi_post = xi_prio + K*(m-C*xi_prio);
P_post = (eye(size(P_prio,1))-K*C)*P_prio*(eye(size(P_prio,1))-K*C)'+K*R*K';
